simulink model "basic_flight_model"  (R2025a)
settings: Solver=VariableStepAuto  StartTime=0.0  StopTime=40  RelTol=1e-3
libraries: aerolibanim x1, aerolibanimutils x1
settings Model: Creator=Josh Fernandez  LastModifiedBy=Josh Fernandez

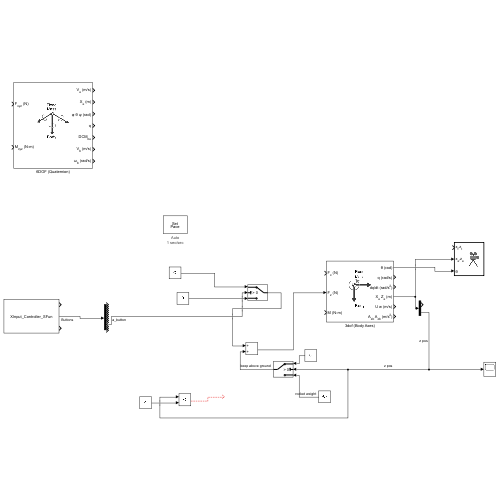
[thumbnail: Simulink's stored preview of the top-level diagram]
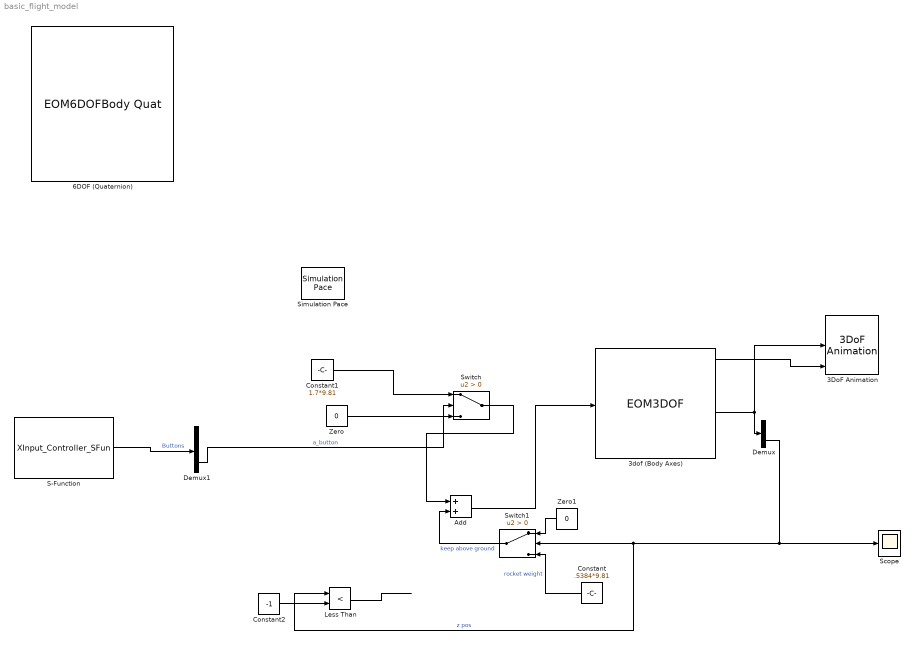
== system basic_flight_model ==
  3DoF Animation : aerolibanim/3DoF Animation  u1=[0 5000 -2000 2000 -5050 -3050]  u2=0.05  u3=1.0  u5=Fixed position  u6=[2000 500 -3150]  u7=10  u8=on
  3dof (Body Axes) : EOM3DOF  v_ini=0  mass=.5384  Iyy=0.0474627  g=-9.81
  6DOF (Quaternion) : EOM6DOFBodyQuat
  Add : Sum
  Constant : Constant  Value=.5384*9.81
  Constant1 : Constant  Value=1.7*9.81
  Constant2 : Constant  Value=-1
  Demux : Demux  Outputs=2
  Demux1 : Demux  Outputs=14
  Less Than : RelationalOperator  Operator=<  OutDataTypeStr=boolean  RndMeth=Simplest  InputSameDT=off
  S-Function : S-Function  FunctionName=XInput_Controller_SFun  Parameters=1  SFunctionDeploymentMode=off  EnableBusSupport=off
  Scope : Scope
      settings: ActiveDisplayYMinimum=-71.398592272865784  ActiveDisplayYMaximum=68.694424376156334
  Simulation Pace : aerolibanimutils/Simulation Pace  SimulationPace=1  SleepMode=Auto  OutputPaceError=off  SampleTime=1/30
  Switch : Switch  Criteria=u2 > Threshold  SaturateOnIntegerOverflow=off  InputSameDT=off
  Switch1 : Switch  Criteria=u2 > Threshold  SaturateOnIntegerOverflow=off  InputSameDT=off
  Zero : Constant  Value=0  OutDataTypeStr=Inherit: Inherit via back propagation
  Zero1 : Constant  Value=0  OutDataTypeStr=Inherit: Inherit via back propagation
  wires:
  3dof (Body Axes)/4 -> 3DoF Animation/2, Demux/1
  Switch/1 -> Add/1
  Demux/2 -> Less Than/1, Switch1/2, Scope/1  "z pos"
  Demux1/11 -> Switch/2  "a_button"
  S-Function/2 -> Demux1/1  "Buttons"
  Constant1/1 -> Switch/1
  Zero/1 -> Switch/3
  Zero1/1 -> Switch1/1
  Switch1/1 -> Add/2  "keep above ground"
  Add/1 -> 3dof (Body Axes)/2
  Constant/1 -> Switch1/3  "rocket weight"
  Constant2/1 -> Less Than/2
  Less Than/1 -> ?
  3dof (Body Axes)/1 -> 3DoF Animation/3
